simulink model "c8mcaputos"  (R2022a)
settings: Solver=ode45  StartTime=0.001  StopTime=1  RelTol=1e-9  EnableMultiTasking=on
PreLoadFcn:
  | ww=[1e-4 1e4]; N=11;
settings Model: Creator=toshiba  LastModifiedBy=xuedi
settings SolverCC: AlgebraicLoopSolver=TrustRegion
settings DataIOCC: LimitDataPoints=on  SaveFormat=Array  SignalLoggingSaveFormat=ModelDataLogs  ReturnWorkspaceOutputs=off
settings OptimizationCC: ExpressionDepthLimit=2147483647  LifeSpan=inf
settings DebuggingCC: UnderspecifiedInitializationDetection=Classic  MergeDetectMultiDrivingBlocksExec=none  SolverPrmCheckMsg=warning  FcnCallInpInsideContextMsg=warning  UnconnectedInputMsg=warning  UnconnectedOutputMsg=warning  UnconnectedLineMsg=warning  AllowSymbolicDim=off  StateNameClashWarn=warning  SFUnexpectedBacktrackingDiag=warning  SFNoUnconditionalDefaultTransitionDiag=warning  SFExecutionAtInitializationDiag=none  SFMachineParentedDataDiag=warning  ArithmeticOperatorsInVariantConditions=warning
settings HardwareCC: ProdBitPerPointer=32  ProdBitPerSizeT=32  ProdBitPerPtrDiffT=32  ProdLargestAtomicFloat=None  ProdIntDivRoundTo=Undefined  ProdEndianess=Unspecified  ProdWordSize=32  ProdHWDeviceType=32-bit Generic
settings ModelReferenceCC: PropagateSignalLabelsOutOfModel=off
settings SFSimCC: SimUseLocalCustomCode=off  CustomCodeUndefinedFunction=UseInterfaceOnly
settings RTWCC: RTWUseLocalCustomCode=off
settings CodeAppCC: StateflowObjectComments=on
settings GRTTargetCC: TargetLangStandard=C89/C90 (ANSI)  CombineOutputUpdateFcns=off  GRTInterface=on
settings ConfigComp: CovMetricSettings=dw  CovSaveCumulativeToWorkspaceVar=on  CovSaveSingleToWorkspaceVar=on  CovExternalEMLEnable=off

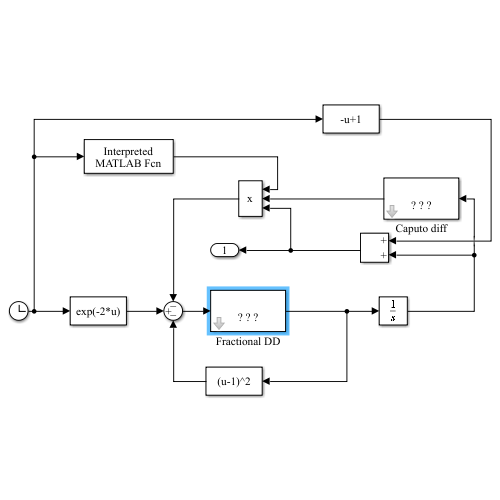
[thumbnail: Simulink's stored preview of the top-level diagram]
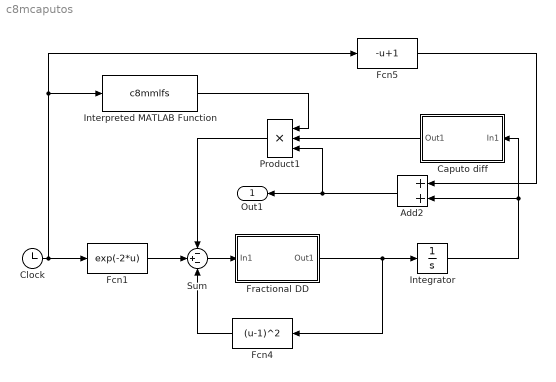
== system c8mcaputos ==
  Add2 : Sum
  Caputo diff : Subsystem  mask{gam=0.555, ww=ww, n=N, y0=[1 -1], kF1=on, kF=Oustaloup filter}
      mask prompts: gam "Derivative order gamma"; ww "Frequency range [wb,wh]"; n "Apprixmation order"; y0 "Initial value"; kF1 "Is a low-pass filter required?"; kF "Filter type"
      mask init:
      | wb=ww(1); wh=ww(2);
      | if kF==1, G=ousta_fod(gam,n,wb,wh);
      | else, G=new_fod(gam,n,wb,wh); end
      | num=G.num{1}; den=G.den{1}; T=1/wh;
      | if kF1==1, den=conv(den,[T,1]); end
      | nam=get_param(gcs,'Name'); q=length(y0); S=''; ngam=ceil(gam);
      | for i=ngam+1:q
      |    astr=num2str(i-1-gam); a1=num2str(y0(i)/gamma(i-gam));
      |    S=[S num2str(a1) '*u^(' astr ')+'];
      | end,
      | S=S(1:end-1); S=strrep(strrep(S,'--','-'),'+-','-');
      | set_param([nam '/Caputo diff/Fcn'],'Expr',S);
      | str=['Caputo\n Der s^' num2str(gam)];
      mask TypeOptions kF: Oustaloup filter | Modified Oustaloup filter
      mask Display: disp(str)
  Clock : Clock
  Fcn1 : Fcn  Expr=exp(-2*u)
  Fcn4 : Fcn  Expr=(u-1)^2
  Fcn5 : Fcn  Expr=-u+1
  Fractional DD : Subsystem  mask{gam=-0.455, ww=ww, n=N, kF1=on, kF=Oustaloup filter}
      mask prompts: gam "Derivative order gamma"; ww "Frequency range [wb,wh]"; n "Apprixmation order"; kF1 "Is a low-pass filter required?"; kF "Filter type"
      mask init:
      | wb=ww(1); wh=ww(2); 
      | if kF==1, G=ousta_fod(gam,n,wb,wh);
      | else, G=new_fod(gam,n,wb,wh); end
      | num=G.num{1}; den=G.den{1}; T=1/wh; str='Fractional\n';
      | if isnumeric(gam)
      | 	if gam>0, str=[str, 'Der  s^' num2str(gam) ];
      | 	else, str=[str, 'Int  s^{' num2str(gam) '}']; end
      | else, str=[str, 'Der  s^gam']; end
      | if kF1==1, G=G*tf(1,[T 1]); end
      mask TypeOptions kF: Oustaloup filter | Modified Oustaloup filter
      mask Display: disp(str)
  Integrator : Integrator
  Interpreted MATLAB Function : MATLABFcn  MATLABFcn=c8mmlfs
  Product1 : Product  Inputs=3  RndMeth=Zero
  Sum : Sum  Inputs=-+-
  Out1 : Outport
  wires:
  Fcn1/1 -> Sum/2
  Product1/1 -> Sum/1
  Clock/1 -> Fcn1/1, Fcn5/1, Interpreted MATLAB Function/1
  Fcn4/1 -> Sum/3
  Add2/1 -> Product1/3, Out1/1
  Fcn5/1 -> Add2/1
  Sum/1 -> Fractional DD/1(In1)
  Integrator/1 -> Caputo diff/1(In1), Add2/2
  Caputo diff/1(Out1) -> Product1/2
  Fractional DD/1(Out1) -> Integrator/1, Fcn4/1
  Interpreted MATLAB Function/1 -> Product1/1

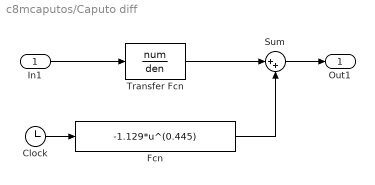
== system c8mcaputos/Caputo diff ==
  In1 : Inport
  Clock : Clock
  Fcn : Fcn  Expr=-1.129*u^(0.445)
  Sum : Sum  Inputs=|++
  Transfer Fcn : TransferFcn  Numerator=num  Denominator=den
  Out1 : Outport
  wires:
  Clock/1 -> Fcn/1
  Transfer Fcn/1 -> Sum/1
  Sum/1 -> Out1/1
  In1/1 -> Transfer Fcn/1
  Fcn/1 -> Sum/2

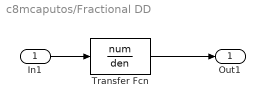
== system c8mcaputos/Fractional DD ==
  In1 : Inport
  Transfer Fcn : TransferFcn  Numerator=num  Denominator=den
  Out1 : Outport
  wires:
  Transfer Fcn/1 -> Out1/1
  In1/1 -> Transfer Fcn/1
